simulink model "DCM_16_Series_Field_For_Spin_Up"  (R2019b)
settings: Solver=VariableStepAuto  StartTime=0.0  StopTime=3000  RelTol=1e-3
model workspace (MAT data in the model file):
  Laf = 0.016
  Rarm = 0.0096
  angular_vel = 0
  angular_vel_13 = 163.55
  angular_vel_14 = 163.55
  angular_vel_15 = 163.55
  angular_vel_16 = 163.55
  angular_vel_2 = 165
  cf = 0.135
  vf = 0.135
libraries: powerlib x22
settings Model: Creator=Sy2  LastModifiedBy=Sy2
settings SolverCC: ZeroCrossAlgorithm=Adaptive
settings DebuggingCC: IgnoredZcDiagnostic=none

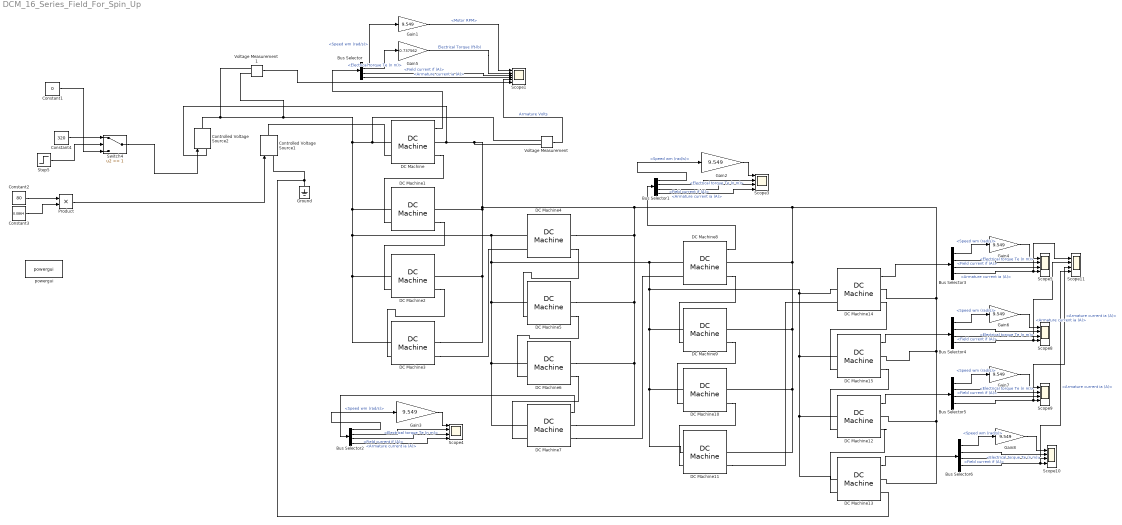
== system DCM_16_Series_Field_For_Spin_Up ==
  Bus Selector{,1..6} (7 alike) : BusSelector  OutputSignals=Speed wm (rad/s),Electrical torque Te (n m),Field current if (A),Armature current ia (A)
  Constant1 : Constant  Value=0
  Constant2 : Constant  Value=80
  Constant3 : Constant  Value=0.0864
  Constant4 : Constant  Value=320
  Controlled Voltage Source1 : powerlib/Electrical Sources/Controlled Voltage Source  Initialize=on  Source_Type=DC  Amplitude=0  Phase=0  Frequency=0  Measurements=Voltage
      settings: SourceProductName=Simscape Electrical
  Controlled Voltage Source2 : powerlib/Electrical Sources/Controlled Voltage Source  Initialize=on  Source_Type=DC  Amplitude=0  Phase=0  Frequency=0  Measurements=Voltage
      settings: SourceProductName=Simscape Electrical
  DC Machine{,1..15} (16 alike) : powerlib/Machines/DC Machine  PresetModel=No  MechanicalLoad=Torque TL  FieldType=Wound  ShowDetailedParameters=on  MeasurementBus=off  RLa="[Rarm  0.002]"  RLf=[0.0054 0.0125]  Laf=Laf  MachineConstant=Torque constant (N.m/A)  Ke=1.8  Kt=1.8  J=137  Bm=vf  Tf=cf  w0=angular_vel  Ifinit=0  TsPowergui=0  TsBlock=-1
      settings: SourceProductName=Simscape Electrical
  Gain{1..4,6..8} (7 alike) : Gain  Gain=9.549
  Gain5 : Gain  Gain=0.737562
  Ground : powerlib/Elements/Ground  LConnTagsString=a
      settings: SourceProductName=Simscape Electrical
  Product : Product
  Scope1 : Scope  NumInputPorts=6
  Scope{3..5,8..11} (7 alike) : Scope  NumInputPorts=4
  Step5 : Step  Time=13  SampleTime=0  VectorParams1D=off  ZeroCross=off
  Switch4 : Switch  Threshold=1  ZeroCross=off
  Voltage Measurement : powerlib/Measurements/Voltage Measurement  PhasorSimulation=off  OutputType=Complex  PSBequivalent=0
      settings: SourceProductName=Simscape Electrical
  Voltage Measurement1 : powerlib/Measurements/Voltage Measurement  PhasorSimulation=off  OutputType=Complex  PSBequivalent=0
      settings: SourceProductName=Simscape Electrical
  powergui : powerlib/powergui  Priority=1  SimulationMode=Continuous  SampleTime=50e-6  frequency=60  Iterations=50  frequencyindice=0  Pbase=100e6  ErrMax=1e-4  UnitsV=kV  UnitsW=MW  buscounter=0  FunctionMessages=off  echomessages=off  EnableUseOfTLC=off  CurrentSourceSwitches=off  DisableSnubberDevices=off  DisableRonSwitches=off  DisableVfSwitches=off  DisplayEquations=off  AutomaticDiscreteSolvers=off  SolverType=Tustin/Backward Euler (TBE)  Interpol=off  ExternalGateDelay=off  methode=off  Ts=100  x0status=blocks  SPID=on  SwTol=0  HookPort=off  NonlinearTolerance=1e-4  nMaxIteration=100  ContinueOnMaxIteration=off  RestoreLinks=warning  ResistiveCurrentMeasurement=off  Frange=[0:2:500]  Ylog=off  Xlog=on  ShowGrid=off  save=off  variable=ZData  structure=0  ZoomFFT=off  StartTime=0.0  cycles=1  DisplayStyle=1  fundamental=60  FreqAxis=off  MaxFrequency=1000  frequencyindicesteady=1  RmsSteady=1  display=off
      settings: SourceProductName=Simscape Electrical
  wires:
  DC Machine/1 -> Bus Selector/1
  Bus Selector/1 -> Gain1/1  "<Speed wm (rad/s)>"
  Bus Selector/3 -> Scope1/3  "<Field current if (A)>"
  Bus Selector/4 -> Scope1/4  "<Armature current ia (A)>"
  Gain1/1 -> Scope1/1  "<Motor RPM>"
  DC Machine8/1 -> Bus Selector1/1
  Bus Selector1/4 -> Scope3/4  "<Armature current ia (A)>"
  Bus Selector1/1 -> Gain2/1  "<Speed wm (rad/s)>"
  Bus Selector1/2 -> Scope3/2  "<Electrical torque Te (n m)>"
  Gain2/1 -> Scope3/1
  Bus Selector1/3 -> Scope3/3  "<Field current if (A)>"
  Bus Selector2/4 -> Scope4/4  "<Armature current ia (A)>"
  Bus Selector2/2 -> Scope4/2  "<Electrical torque Te (n m)>"
  Gain3/1 -> Scope4/1
  Bus Selector2/3 -> Scope4/3  "<Field current if (A)>"
  DC Machine7/1 -> Bus Selector2/1
  Bus Selector2/1 -> Gain3/1  "<Speed wm (rad/s)>"
  Constant2/1 -> Product/1
  Bus Selector/2 -> Gain5/1  "<Electrical torque Te (n m)>"
  Gain5/1 -> Scope1/2  "Electrical Torque (ft-lb)"
  Constant3/1 -> Product/2
  Gain6/1 -> Scope8/1
  DC Machine15/1 -> Bus Selector4/1
  Bus Selector4/4 -> Scope11/2, Scope8/4  "<Armature current ia (A)>"
  Bus Selector4/1 -> Gain6/1  "<Speed wm (rad/s)>"
  Bus Selector4/2 -> Scope8/2  "<Electrical torque Te (n m)>"
  Bus Selector4/3 -> Scope8/3  "<Field current if (A)>"
  Bus Selector5/3 -> Scope9/3  "<Field current if (A)>"
  DC Machine12/1 -> Bus Selector5/1
  Gain7/1 -> Scope9/1
  Bus Selector5/2 -> Scope9/2  "<Electrical torque Te (n m)>"
  Bus Selector5/1 -> Gain7/1  "<Speed wm (rad/s)>"
  Bus Selector5/4 -> Scope11/3, Scope9/4  "<Armature current ia (A)>"
  Bus Selector6/4 -> Scope11/4, Scope10/4  "<Armature current ia (A)>"
  Gain8/1 -> Scope10/1
  Bus Selector6/1 -> Gain8/1  "<Speed wm (rad/s)>"
  Bus Selector6/2 -> Scope10/2  "<Electrical torque Te (n m)>"
  Bus Selector6/3 -> Scope10/3  "<Field current if (A)>"
  DC Machine13/1 -> Bus Selector6/1
  Bus Selector3/3 -> Scope5/3  "<Field current if (A)>"
  DC Machine14/1 -> Bus Selector3/1
  Gain4/1 -> Scope5/1
  Bus Selector3/2 -> Scope5/2  "<Electrical torque Te (n m)>"
  Bus Selector3/1 -> Gain4/1  "<Speed wm (rad/s)>"
  Bus Selector3/4 -> Scope11/1, Scope5/4  "<Armature current ia (A)>"
  Product/1 -> Controlled Voltage Source1/1
  Constant4/1 -> Switch4/1
  Constant1/1 -> Switch4/3
  Switch4/1 -> Controlled Voltage Source2/1
  Step5/1 -> Switch4/2
  Voltage Measurement/1 -> Scope1/5  "Armature Volts"
  Voltage Measurement1/1 -> Scope1/6
  connections:
  DC Machine/RConn2 -- DC Machine1/LConn2
  DC Machine1/RConn2 -- DC Machine2/LConn2
  DC Machine2/RConn2 -- DC Machine3/LConn2
  DC Machine3/RConn2 -- DC Machine4/LConn2
  DC Machine4/RConn2 -- DC Machine5/LConn2
  DC Machine5/RConn2 -- DC Machine6/LConn2
  DC Machine6/RConn2 -- DC Machine7/LConn2
  DC Machine7/RConn2 -- DC Machine8/LConn2
  DC Machine8/RConn2 -- DC Machine9/LConn2
  DC Machine9/RConn2 -- DC Machine10/LConn2
  DC Machine10/RConn2 -- DC Machine11/LConn2
  DC Machine11/RConn2 -- DC Machine14/LConn2
  DC Machine14/RConn2 -- DC Machine15/LConn2
  DC Machine15/RConn2 -- DC Machine12/LConn2
  DC Machine12/RConn2 -- DC Machine13/LConn2
  DC Machine/LConn2 -- Controlled Voltage Source1/RConn1
  Ground/LConn1 -- DC Machine13/RConn2 -- Controlled Voltage Source1/LConn1
  Controlled Voltage Source2/RConn1 -- DC Machine14/LConn1 -- DC Machine15/LConn1 -- DC Machine13/LConn1 -- DC Machine12/LConn1 -- DC Machine9/LConn1 -- DC Machine10/LConn1 -- DC Machine11/LConn1 -- DC Machine8/LConn1 -- DC Machine5/LConn1 -- DC Machine7/LConn1 -- DC Machine6/LConn1 -- DC Machine4/LConn1 -- DC Machine3/LConn1 -- DC Machine2/LConn1 -- DC Machine1/LConn1 -- Voltage Measurement/LConn1 -- DC Machine/LConn1 -- Voltage Measurement1/LConn2 -- Voltage Measurement1/LConn1
  DC Machine12/RConn1 -- DC Machine13/RConn1 -- DC Machine15/RConn1 -- DC Machine14/RConn1 -- Voltage Measurement/LConn2 -- Controlled Voltage Source2/LConn1 -- DC Machine/RConn1 -- DC Machine1/RConn1 -- DC Machine2/RConn1 -- DC Machine3/RConn1 -- DC Machine4/RConn1 -- DC Machine5/RConn1 -- DC Machine7/RConn1 -- DC Machine6/RConn1 -- DC Machine8/RConn1 -- DC Machine9/RConn1 -- DC Machine11/RConn1 -- DC Machine10/RConn1
